simulink library "pixhawk_slib_misc_utils"  (R2017b)
settings: Solver=ode45  StartTime=0.0  StopTime=10.0  RelTol=1e-3
Description:
  | pixhawk_slib_misc_utils library
  | 
  | Pixhawk PSP library for miscellaneous blocks.
settings Model: Creator=skuznick  LastModifiedBy=dream
settings DataIOCC: LimitDataPoints=on  SaveFormat=Array
settings OptimizationCC: BlockReduction=off  BooleanDataType=off  LifeSpan=inf
settings DebuggingCC: SaveWithParameterizedLinksMsg=none  UnderspecifiedInitializationDetection=Classic  MergeDetectMultiDrivingBlocksExec=none  SignalResolutionControl=TryResolveAllWithWarning  AllowSymbolicDim=off  StrictBusMsg=Warning  SFUnexpectedBacktrackingDiag=warning  SFNoUnconditionalDefaultTransitionDiag=warning  SFExecutionAtInitializationDiag=none
settings HardwareCC: ProdBitPerPointer=32  ProdBitPerSizeT=32  ProdBitPerPtrDiffT=32  ProdLargestAtomicFloat=None  ProdIntDivRoundTo=Undefined  ProdEndianess=Unspecified  ProdWordSize=32  ProdHWDeviceType=32-bit Generic  TargetUnknown=on
settings ModelReferenceCC: PropagateSignalLabelsOutOfModel=off
settings CodeAppCC: StateflowObjectComments=on
settings GRTTargetCC: TargetLangStandard=C89/C90 (ANSI)  GeneratePreprocessorConditionals=Disable all
settings ConfigComp: CovMetricSettings=dw  CovHtmlReporting=on  CovSaveCumulativeToWorkspaceVar=on  CovSaveSingleToWorkspaceVar=on  CovExternalEMLEnable=off  CovSFcnEnable=off

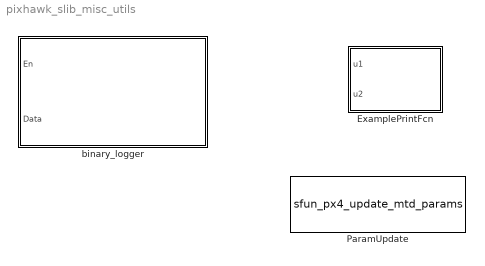
== system pixhawk_slib_misc_utils ==
  ExamplePrintFcn : MATLAB Function  Description=|  TreatAsAtomicUnit=on
      | Example MATLAB block for printing out to terminal.
      | 
      | Use this as a way to output strings to the shell window for debugging/status purposes.
      mask help:
      | ExamplePrintFcn
      |
      | Shows an example of a printf function using coder.ceval.
  ParamUpdate : S-Function  Description=|  FunctionName=sfun_px4_update_mtd_params  Parameters='differential_pressure',TLC_StrSet,NumParams,Ts  SFunctionDeploymentMode=off  EnableBusSupport=off  SFcnStateName=uORB_fd  mask{Unformatted_StrSet=0, TLC_StrSet=0, NumParams=0, Ts=0}
      | ParamUpdate Block
      | 
      | Use this block at your top-level of your model to insert a "parameter update" function in the generated code.
      mask help:
      | Parameter Update
      |
      | Use this block at the top-level to insert code into the source that checks for parameter updated values.
      mask init:
      | % A structure of data can be stored in the block UserData
      | maskData = get_param(gcb,'UserData');
      | 
      | % Block Param formatted string
      | if isfield(maskData,'Unformated_StrSet')
      |     Unformatted_StrSet = maskData.Unformatted_StrSet;
      | else
      |     Unformatted_StrSet = {'<unformatted_placeholder_param>'};
      | end
      | 
      | % TLC formatted string
      | if isfield(maskData,'TLC_StrSet')
      |     TLC_StrSet = maskData.TLC_StrSet;
      | else
      |     TLC_StrSet = {'["<unformatted_placeholder_param>"]'};
      | end
      | 
      | % NumParams
      | if isfield(maskData,'NumParams')
      |     NumParams =  maskData.NumParams;
      | else
      |     NumParams = 1;
      | end
      | 
      | % Sample-time
      | if isfield(maskData,'Ts') 
      |     try
      |         Ts = evalin('base',maskData.Ts);
      |     catch
      |         Ts = -1;
      |     end
      | else
      |     Ts = -1;
      | end
      | 
      | %Uncomment these lines to temporarily set these with initial values
      | % maskData.Unformatted_StrSet = {''}
      | % maskData.TLC_StrSet = ''
      | % maskData.NumParams = 1
      | % maskData.Ts = '-1';
      | % 
      | % set_param(gcb,'UserData',maskData)
      | % set_param(gcb, 'UserDataPersistent', 'on');
      | % 
      | % S-Function expects the parameters to be passed in as so:
      | % char_array = ["name1","name2"]
      settings: DestroyFcn=Pixhawk_CSC.BlockParamUpdate.ParamUpdateMaskDialog(gcbh,bdroot,'Delete');  OpenFcn=Pixhawk_CSC.BlockParamUpdate.ParamUpdateMaskDialog(gcbh,bdroot,'Open');  SFcnIsStateOwnerBlock=on
      mask Help: eval('sharedhelp(''ParamUpdate'')');
      mask Display: disp('Parameter Update module')
  binary_logger : Subsystem  Description=|  mask(Pixhawk Binary Logger){logfile=/fs/microsd/log/2024-09-20, cacheflag=on, isUlg=off, numRecs=1000}
      | Binary Logger Block (MATLAB block)
      | 
      | Log a vector of data to a file on the SD card. The first enable port must trigger high and then low during the execution of the program for a successful write to disk space. 
      | If the enable port does not fall low before the generated code is finished executing the file will be still considered ‘open’ and not accessible. 
      | In order for proper SD card data writing ensure that the above directory path points to some place in /fs/microsd/ 
      |   
      | The data input can be a vector signal concatenated together to allow for multiple signal logging. 
      |   
      | Note that an example file has been provided to showcase data logging and reading/extraction. 
      | Under the examples look for px4demo_log.slx to see how one can implement a logging block and use the readdata.m function to the logged data on the SD card. 
      | 
      | Processing Captured Log File 
      | In order to process the binary log file there is a convenient MATLAB function provided. 
      | A function px4_read_binary_file has been added to the MATLAB path which is used to read in binary files and display the data. 
      | The function expects one input argument which is the name of the binary log file (in single quotes).  It return a data vector and number of records read from the file.
      | 
      | %% Load the data into MATLAB from a binary log file
      | % Usage: >> [datapoints, numpoints] = px4_read_binary_file('datafile.log')
      | % Header information format:
      | %           String "MWLOGV##"
      | %           Time/Date 4 bytes (time())
      | %           Number of Signals per record Logged 1 bytes (256 max)
      | %           Data Type of Signals Logged  1 bytes (1-10)
      | %           Number of bytes per record 2 (65535 max)
      | % Plot Data Example: plot([1:numpoints], datapoints(1,:), [1:numpoints], datapoints(2,:))
      mask prompts: cacheflag "Cache in Memory"; isUlg "Use .ulg suffix"; numRecs "Max Record Count"
      mask help:
      | Log a vector of data to a file on the SD card
      |
      | If Cache in Memory is on data is written when en goes low or when max number of records specified is reached.
      | Otherwise Max Number of Records is used to indicate when to performa an fflush out to file.
      mask init:
      | logname=uint8(logfile);
      mask Help: eval('sharedhelp(''binary_logger'')');
      mask Display:
      | fprintf(get_param(gcb,'logfile'))
      | port_label('input',1,'en')
      | port_label('input',2,'data')

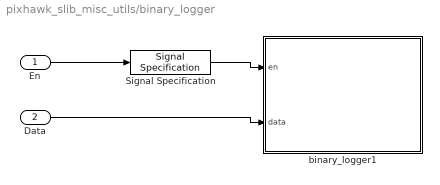
== system pixhawk_slib_misc_utils/binary_logger ==
  En : Inport
  Data : Inport  Port=2
  Signal Specification : SignalSpecification  OutDataTypeStr=boolean
  binary_logger1 : MATLAB Function  TreatAsAtomicUnit=on
  wires:
  Signal Specification/1 -> binary_logger1/1(en)
  En/1 -> Signal Specification/1
  Data/1 -> binary_logger1/2(data)

== matlab function pixhawk_slib_misc_utils/binary_logger/binary_logger1 ==
  data: en input boolean; data input; logname parameter uint8; cacheflag parameter boolean; numRecs parameter uint32; isUlg parameter boolean
%% Binary Logger
% Note: All data needs to be of the same type (e.g. double)
% Header information format:
%           String "MWLOGV##"
%           Time/Date 4 bytes (time())
%           Number of Signals per record Logged 1 byte (256 max)
%           Data Type of Signals Logged  1 byte (1-10)
%           Number of bytes per record 2 bytes (65535 max)
% This does NOT include the number of data sets logged.  
% i.e. The Reader is responsible for reading until EOF.
% MathWorks Pilot Engineering 2015
% Steve Kuznicki
function binary_logger(en, data, logname, cacheflag, numRecs, isUlg)
%#codegen
    persistent fp isflushed isopen count lognumstr elem_size vect_size datastore
    coder.cinclude('<stdio.h>');
    coder.cinclude('<time.h>');
    coder.cinclude('<sys/stat.h>');

    if isempty(count)
        count = uint32(0);
        if isUlg
            lognumstr = 0;
        else
            lognumstr = 65;
        end
        
        isopen = false;
        fp = coder.opaque('FILE*', 'NULL');
        isflushed = false;
        elem_size = uint16(1);
        vect_size = coder.const(uint8(numel(data)));
        if cacheflag == true
            datastore = zeros(numRecs*uint32(coder.const(numel(data))), 1, 'like', data);
        end
    end

    if (en)
        if isopen == false
            [elsize, eltype] = get_elem_size(data);
            elem_size = coder.const(uint16(elsize));
            elem_type = coder.const(uint8(eltype));
            vect_size = coder.const(uint8(numel(data)));
            if isUlg
                myNum=lognumstr;
                L0=mod(myNum,10)+48;
                myNum=floor(myNum/10);
                L1=mod(myNum,10)+48;
                myNum=floor(myNum/10);
                L2=mod(myNum,10)+48;
                myNum=floor(myNum/10);
                L3=mod(myNum,10)+48;
                myNum=floor(myNum/10);
                L4=mod(myNum,10)+48;
                myNum=floor(myNum/10);
                L5=mod(myNum,10)+48;
                coder.ceval('printf',['OPENING file %s vect_size %d elem_size %d numRecs %d %c' uint8(0)], ...
                    [logname, '/', char(L5),char(L4),'-', char(L3),char(L2),'-', char(L1),char(L0), '.ulg', int8(0)], uint32(vect_size), uint32(elem_size), uint32(numRecs), uint8(10));
                coder.ceval('mkdir',[logname, int8(0)],0777);
                fp = coder.ceval('fopen',  [logname, '/', char(L5),char(L4),'-', char(L3),char(L2),'-', char(L1),char(L0), '.ulg', int8(0)], ['wb', int8(0)]);
            else
                coder.ceval('printf',['OPENING file %s vect_size %d elem_size %d numRecs %d %c' uint8(0)], ...
                    [logname, '_', char(lognumstr), '.bin', int8(0)], uint32(vect_size), uint32(elem_size), uint32(numRecs), uint8(10));
                fp = coder.ceval('fopen', [logname, '_', char(lognumstr), '.bin', int8(0)], ['wb', int8(0)]);
            end

            lognumstr = lognumstr + 1;
            isflushed = false;
            count = uint32(0);
            isopen = true;
            % Write header information here
            % header token + version
            mlStrVer = 'MWLOGV01';
            coder.ceval('fwrite', coder.rref(mlStrVer), uint32(1), length(mlStrVer), fp);
            % date/time
            tm = uint32(0);
            tmptr = uint32(0);
            tm = coder.ceval('time',coder.wref(tmptr));
            coder.ceval('fwrite', coder.rref(tm), uint32(4), uint32(1), fp);
            % number of elements in each record
            coder.ceval('fwrite', coder.rref(vect_size), uint32(1), uint32(1), fp);
            % data type of the elements
            coder.ceval('fwrite', coder.rref(elem_type), uint32(1), uint32(1), fp);
            % size of each record in bytes
            recSize = elem_size * uint16(vect_size);
            coder.ceval('fwrite', coder.rref(recSize), uint32(2), uint32(1), fp);
        end
        % cache data in memory or use fwrite
        if cacheflag == true
            addr = (count*uint32(vect_size))+1;
            for idx = 1:vect_size
                datastore(addr) = data(idx);
                addr = addr + 1;
            end
        else
            coder.ceval('fwrite', coder.rref(data), elem_size, vect_size, fp);
        end
        count = count + uint32(1);
        % check for data count limit
        if count >= numRecs
            if cacheflag
                for idx = 1:count*uint32(vect_size)
                    coder.ceval('fwrite', coder.rref(datastore(idx)), elem_size, uint32(1), fp);
                end
            end
            coder.ceval('fflush', fp);
            isflushed = false;
            count = uint32(0);
        end
    else
        if isopen == true
            if ~isflushed
                coder.ceval('printf',['CLOSING file. count = %d %c' uint8(0)], uint32(count), uint8(10));
                if cacheflag
                    count = count + uint32(1);
                    for idx = 1:count*uint32(vect_size)
                        coder.ceval('fwrite', coder.rref(datastore(idx)), elem_size, uint32(1), fp);
                    end
                end
                coder.ceval('fflush', fp);
                isflushed = true;
            end
            coder.ceval('fclose', fp);
        end
        isopen = false;
        count = uint32(0);
    end
end

% return the size of the element in bytes
function [elem_size, dtype] = get_elem_size(data)
    switch(class(data))
        case 'double'
            elem_size = 8;
            dtype = 1;
        case 'single'
            elem_size = 4;
            dtype = 2;
        case 'int32'
            elem_size = 4;
            dtype = 3;
        case 'uint32'
            elem_size = 4;
            dtype = 4;
        case 'int16'
            elem_size = 2;
            dtype = 5;
        case 'uint16'
            elem_size = 2;
            dtype = 6;
        case 'int8'
            elem_size = 1;
            dtype = 7;
        case 'uint8'
            elem_size = 1;
            dtype = 8;
        case 'logical'
            elem_size = 1;
            dtype = 9;
        case 'embedded.fi'
            nt = numerictype(data);
            elem_size = 2^ceil(log2(ceil(nt.WordLength / 8)));
            dtype = 10;
    end
    if ~isreal(data)
        elem_size = elem_size*2;
    end
    
    elem_size = uint16(elem_size);
    dtype = uint8(dtype);
end

== matlab function pixhawk_slib_misc_utils/ExamplePrintFcn ==
  data: u1 input; u2 input
function fcn(u1, u2)
%#codegen

if strcmp(coder.target, 'rtw') == true
    coder.ceval('printf','%d %d %c', int32(u1), int32(u2), int8(10))
end
